simulink model "MotorIdentPos"  (R2013a)
settings: Solver=FixedStepDiscrete  StartTime=0.0  StopTime=Time  FixedStep=0.01  RelTol=1e-3
values from neighbouring files (symbols this model uses):
  joint = CoupledJoints('experiments', 'iCubGenova03', 'torso')    [CoupledExper-IDLE.m]    (also in CoupledExper.m = joint.loadRefFile('ref'); CoupledJoints.m = [joint Motor(date,robotName, part, type,'yaw')]; FrictionTest.m = joint.loadFriction('idle.mat',1); JointStructure.m = struct)
  Reference = struct    [CoupledJoints.m]    (also in ReferenceLoad.m; WBLMotor.m)
libraries: WBCLibrary x8, utility x1
settings Model: Creator=Raffaello  LastModifiedBy=Raffaello
settings DataIOCC: LimitDataPoints=off  OutputSaveName=out

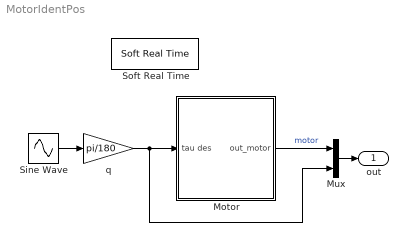
== system MotorIdentPos ==
  Motor : Subsystem
  Mux : Mux  Inputs=2
  Sine Wave : Sin  Amplitude=Reference.sinAmp  Bias=Reference.sinBias  Frequency=Reference.sinFreq*2*pi  SampleTime=0
  Soft Real Time : utility/Soft Real Time  x=1
  q : Gain  Gain=pi/180
  out : Outport
  wires:
  Motor/1(out_motor) -> Mux/1  "motor"
  Mux/1 -> out/1
  Sine Wave/1 -> q/1
  q/1 -> Mux/2, Motor/1(tau des)

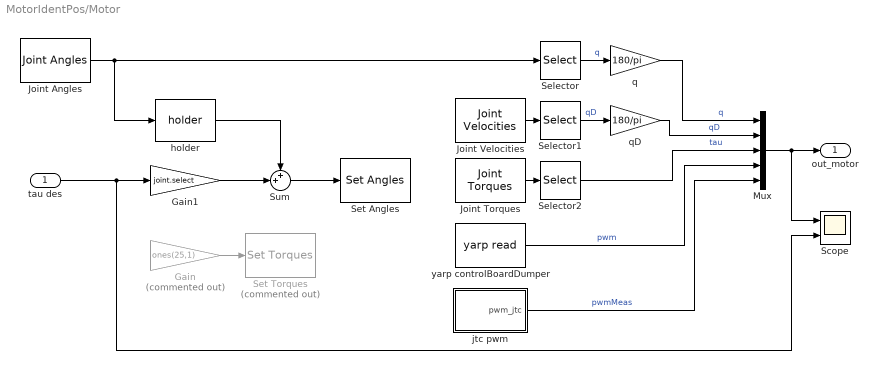
== system MotorIdentPos/Motor ==
  tau des : Inport
  Gain : Gain  Commented=on  Gain=ones(25,1)
  Gain1 : Gain  Gain=joint.select
  Joint Angles : WBCLibrary/wholeBodyStates/Joint Angles  robotName=robotName  localName=localName
  Joint Torques : WBCLibrary/wholeBodyStates/Joint Torques  robotName=robotName  localName=localName
  Joint Velocities : WBCLibrary/wholeBodyStates/Joint Velocities  robotName=robotName  localName=localName
  Mux : Mux  Inputs=5
  Scope : Scope  NumInputPorts=2
      settings: ShowLegends=on  TimeRange=10  YMin=-125~-2  YMax=125~1.5  SaveName=ScopeData2
  Selector : Selector  InputPortWidth=25  IndexOptions=Index vector (dialog)  Indices=[joint.number]  OutputSizes=1
  Selector1 : Selector  InputPortWidth=25  IndexOptions=Index vector (dialog)  Indices=[joint.number]  OutputSizes=1
  Selector2 : Selector  InputPortWidth=25  IndexOptions=Index vector (dialog)  Indices=[joint.number]  OutputSizes=1
  Set Angles : WBCLibrary/wholeBodyActuators/Set Angles  val=5  robotName=robotName  localName=localName
  Set Torques : WBCLibrary/wholeBodyActuators/Set Torques  Commented=on  val=6  robotName=robotName  localName=localName
  Sum : Sum  Inputs=++|
  "holder " : WBCLibrary/Utilities/holder 
  jtc pwm : Subsystem
  q : Gain  Gain=180/pi
  qD : Gain  Gain=180/pi
  yarp controlBoardDumper : WBCLibrary/Utilities/yarp read  from=['/controlBoardDumper/' joint.path '/getOutputs']  to='...'  num=1  blocking=off  timestamp=off
  out_motor : Outport
  wires:
  Gain/1 -> Set Torques/1
  Joint Velocities/1 -> Selector1/1
  Mux/1 -> out_motor/1, Scope/1
  Joint Angles/1 -> "holder "/1, Selector/1
  Joint Torques/1 -> Selector2/1
  yarp controlBoardDumper/1 -> Mux/4  "pwm"
  Selector/1 -> q/1  "q"
  Selector1/1 -> qD/1  "qD"
  Selector2/1 -> Mux/3  "tau"
  q/1 -> Mux/1  "q"
  qD/1 -> Mux/2  "qD"
  jtc pwm/1(pwm_jtc) -> Mux/5  "pwmMeas"
  tau des/1 -> Scope/2, Gain1/1
  Sum/1 -> Set Angles/1
  "holder "/1 -> Sum/1
  Gain1/1 -> Sum/2

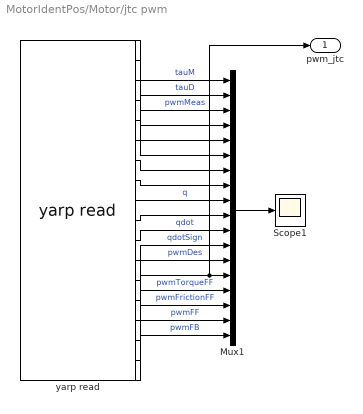
== system MotorIdentPos/Motor/jtc pwm ==
  Mux1 : Mux  Inputs=18
  Scope1 : Scope
      settings: ShowLegends=on
  yarp read : WBCLibrary/Utilities/yarp read  from=['/jtc/monitor:o']  to='...'  num=18  blocking=off  timestamp=off
  pwm_jtc : Outport
  wires:
  yarp read/18 -> Mux1/18  "pwmFB"
  Mux1/1 -> Scope1/1
  yarp read/1 -> Mux1/1  "tauM"
  yarp read/2 -> Mux1/2  "tauD"
  yarp read/3 -> Mux1/3
  yarp read/4 -> Mux1/4
  yarp read/5 -> Mux1/5
  yarp read/10 -> Mux1/10
  yarp read/6 -> Mux1/6
  yarp read/7 -> Mux1/7
  yarp read/8 -> Mux1/8
  yarp read/9 -> Mux1/9  "q"
  yarp read/11 -> Mux1/11  "qdot"
  yarp read/12 -> Mux1/12  "qdotSign"
  yarp read/13 -> Mux1/13  "pwmDes"
  yarp read/14 -> pwm_jtc/1, Mux1/14  "pwmMeas"
  yarp read/15 -> Mux1/15  "pwmTorqueFF"
  yarp read/16 -> Mux1/16  "pwmFrictionFF"
  yarp read/17 -> Mux1/17  "pwmFF"
